simulink model "Properties_Sensor_Primitives"  (R2012b)
settings: Solver=FixedStepDiscrete  StartTime=0.0  StopTime=10.0  FixedStep=0.1  RelTol=1e-3
settings Model: Creator=Kerianne  LastModifiedBy=Kerianne
settings DataIOCC: SaveFormat=Structure
settings OptimizationCC: InlineParams=on

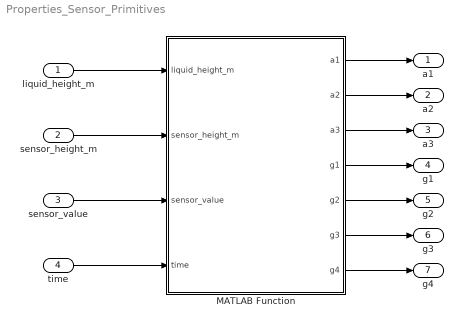
== system Properties_Sensor_Primitives ==
  liquid_height_m : Inport  OutDataTypeStr=double
  sensor_height_m : Inport  Port=2  OutDataTypeStr=double
  sensor_value : Inport  Port=3  OutDataTypeStr=double
  time : Inport  Port=4  OutDataTypeStr=double
  MATLAB Function : MATLAB Function  TreatAsAtomicUnit=on
  a1 : Outport  OutDataTypeStr=boolean
  a2 : Outport  Port=2  OutDataTypeStr=boolean
  a3 : Outport  Port=3  OutDataTypeStr=boolean
  g1 : Outport  Port=4  OutDataTypeStr=boolean
  g2 : Outport  Port=5  OutDataTypeStr=boolean
  g3 : Outport  Port=6  OutDataTypeStr=boolean
  g4 : Outport  Port=7  OutDataTypeStr=boolean
  wires:
  time/1 -> MATLAB Function/4(time)
  liquid_height_m/1 -> MATLAB Function/1(liquid_height_m)
  sensor_height_m/1 -> MATLAB Function/2(sensor_height_m)
  sensor_value/1 -> MATLAB Function/3(sensor_value)
  MATLAB Function/1(a1) -> a1/1
  MATLAB Function/2(a2) -> a2/1
  MATLAB Function/3(a3) -> a3/1
  MATLAB Function/4(g1) -> g1/1
  MATLAB Function/5(g2) -> g2/1
  MATLAB Function/6(g3) -> g3/1
  MATLAB Function/7(g4) -> g4/1

== matlab function Properties_Sensor_Primitives/MATLAB Function ==
  data: a1 output; a2 output; a3 output; liquid_height_m input; g1 output; sensor_height_m input; sensor_value input; time input; g2 output; g3 output; g4 output
function [a1, a2, a3, g1, g2, g3, g4]   = verification_condition(...
    liquid_height_m, sensor_height_m, sensor_value, time)
% Updated 25 Feb 2015
% Assumptions
% assume "Initially the sensor height is greater than the current height" 
a1 = liquid_height_init_cond(liquid_height_m, sensor_height_m, time); 
% assume "the liquid height is non-negative":
a2 = liquid_height_m >= 0.0;
% assume "the sensor height is non-negative":
a3 = sensor_height_m >= 0.0;
		
% Guarantees
% guarantee "If the tank height is greater than or equal to the sensor height then Sensor_Value is true"
g1 = sensor_true(liquid_height_m, sensor_height_m, sensor_value);
% guarantee "If the tank height is less than the sensor height then Sensor_Value is false" 
g2 = sensor_false(liquid_height_m, sensor_height_m, sensor_value);
% guarantee "The sensor should be false initially"
g3 = sensor_init_cond(sensor_value, time);
% guarantee "The sensor_height is the same as the specified sensor height"
g4 = sensor_height_verity(sensor_value);
	
function c = implies(a,b)      
     c = ((not (a)) || b);
     
% a1 
function result = liquid_height_init_cond(liquid_height_m, sensor_height_m, time) 
    UnderThisCondition = (time == 0.0);
    ResultShouldBe = (sensor_height_m > liquid_height_m);
    result = implies(UnderThisCondition, ResultShouldBe);
% g1 "If the tank height is greater than or equal to the sensor height then Sensor_Value is true"
function result = sensor_true(liquid_height_m, sensor_height_m, sensor_value) 
    UnderThisCondition = (liquid_height_m >= sensor_height_m);
    ResultShouldBe = (sensor_value == 1.0);
    result = implies(UnderThisCondition, ResultShouldBe);
% g2 "If the tank height is less than the sensor height then Sensor_Value is false" 
function result = sensor_false(liquid_height_m, sensor_height_m, sensor_value) 
    UnderThisCondition = (liquid_height_m < sensor_height_m);
    ResultShouldBe = (sensor_value == 0.0);
    result = implies(UnderThisCondition, ResultShouldBe);    
% g3 "The sensor should be false initially"
function result = sensor_init_cond(sensor_value, time) 
    UnderThisCondition = (time == 0.0);
    ResultShouldBe = (sensor_value == 0.0);
    result = implies(UnderThisCondition, ResultShouldBe);
% g4 "The sensor_height is the same as the specified sensor height"
function result = sensor_height_verity(sensor_value) 
   result = (sensor_value == sensor_value);
